simulink model "motor_model"  (R2019a)
settings: Solver=VariableStepAuto  StartTime=0.0  StopTime=10.0  RelTol=1e-3
values from neighbouring files (symbols this model uses):
  D = 0.2    [motor.m]    (also in motor_func.m)
  J = 0.5    [motor.m]    (also in motor_func.m)
  K_e = 6.0    (= 6)    [motor.m]    (also in motor_func.m)
  K_tau = 4.0    (= 4)    [motor.m]    (also in motor_feedback.m; motor_func.m)
  L = 0.00034    [motor.m]    (also in motor_func.m)
  R = 0.41    [motor.m]    (also in motor_func.m)
settings Model: Creator=itomasa  LastModifiedBy=itomasa

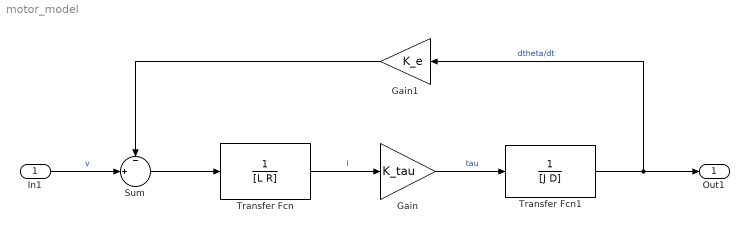
== system motor_model ==
  In1 : Inport
  Gain : Gain  Gain=K_tau
  Gain1 : Gain  Gain=K_e
  Sum : Sum  Inputs=-|+||
  Transfer Fcn : TransferFcn  Denominator=[L R]
  Transfer Fcn1 : TransferFcn  Denominator=[J D]
  Out1 : Outport
  wires:
  Transfer Fcn/1 -> Gain/1  "i"
  Gain/1 -> Transfer Fcn1/1  "tau"
  Transfer Fcn1/1 -> Gain1/1, Out1/1  "dtheta/dt"
  Gain1/1 -> Sum/1
  Sum/1 -> Transfer Fcn/1
  In1/1 -> Sum/2  "v"
